simulink model "PWM-graphique"  (R2024b)
settings: Solver=VariableStepAuto  StartTime=0.0  StopTime=0.02  RelTol=1e-3
libraries: simulink x1
settings Model: Creator=valun  LastModifiedBy=valun

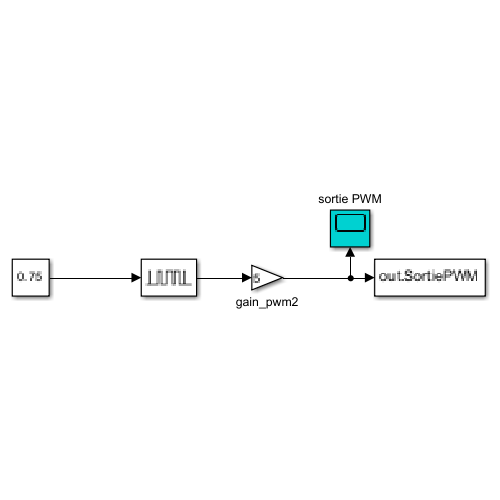
[thumbnail: Simulink's stored preview of the top-level diagram]
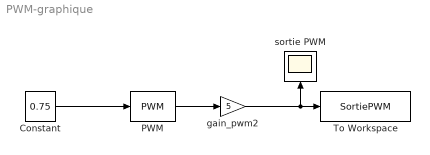
== system PWM-graphique ==
  Constant : Constant  Value=0.75
  PWM : simulink/Discontinuities/PWM  DisableCoverage=on  Period=0.002  InitialDelay=0  DisallowZeroDutyCycle=off  RunAtFixedTimeIntervals=off  SampleTime=0.1
  To Workspace : ToWorkspace  VariableName=SortiePWM  SaveFormat=Timeseries  SampleTime=-1
  gain_pwm2 : Gain  Gain=5
  sortie PWM : Scope
  wires:
  PWM/1 -> gain_pwm2/1
  Constant/1 -> PWM/1
  gain_pwm2/1 -> To Workspace/1, sortie PWM/1
